simulink model "wrksp_integer_sis_"  (R2024a)
settings: Solver=VariableStepAuto  StartTime=0.0  StopTime=0.1  RelTol=1e-3
values from neighbouring files (symbols this model uses):
  A = zeros(n,n)    [ayuda.m]    (also in wrksp_dif_atras.m; wrksp_dif_atras_2.m; wrksp_int_crtl_snd_der.m; wrksp_integrate.m)
  x0 = []    [ayuda.m]    (also in s_fun_sim_auto_center.m = zeros(1,n); s_fun_sim_auto_center_v2.m = [x0_1,x0_2]; s_fun_simultaneo.m = [exp(-100*(l(1)-0.5)^2),exp(-100*(l(2)-0.5)^2) , exp(-100*(l; s_fun_simultaneo_v2.m = [x0_1,x0_2])
settings Model: Creator=omar  LastModifiedBy=omar

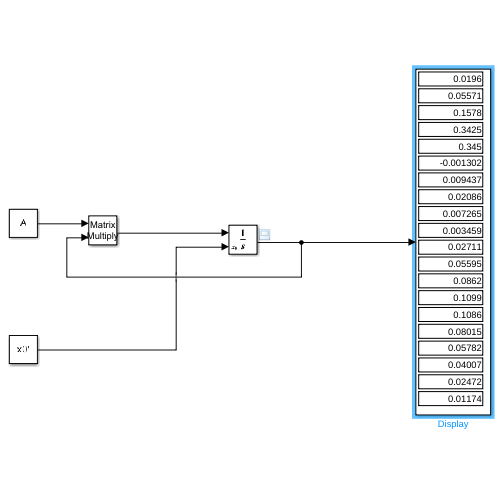
[thumbnail: Simulink's stored preview of the top-level diagram]
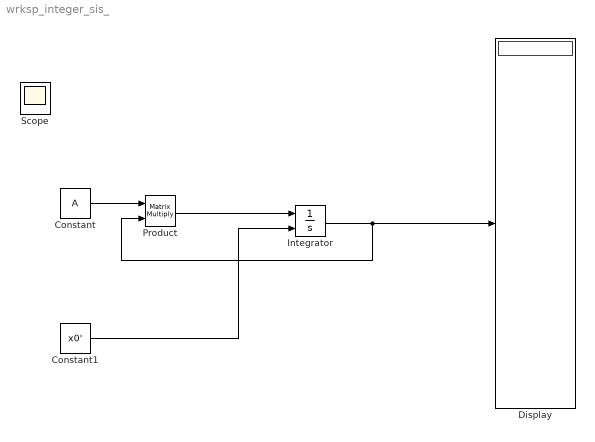
== system wrksp_integer_sis_ ==
  Constant : Constant  Value=A
  Constant1 : Constant  Value=x0'  VectorParams1D=off
  Display : Display
  Integrator : Integrator  InitialConditionSource=external
  Product : Product  Multiplication=Matrix(*)
  Scope : Scope
  wires:
  Constant/1 -> Product/1
  Product/1 -> Integrator/1
  Constant1/1 -> Integrator/2
  Integrator/1 -> Product/2, Display/1
